simulink model "sistemaPIDSin"  (R2024b)
settings: Solver=VariableStepAuto  StartTime=0.0  StopTime=10  RelTol=1e-3
undefined symbols (not defined in the file): step_value, Ts
settings Model: Creator=estel  LastModifiedBy=estel

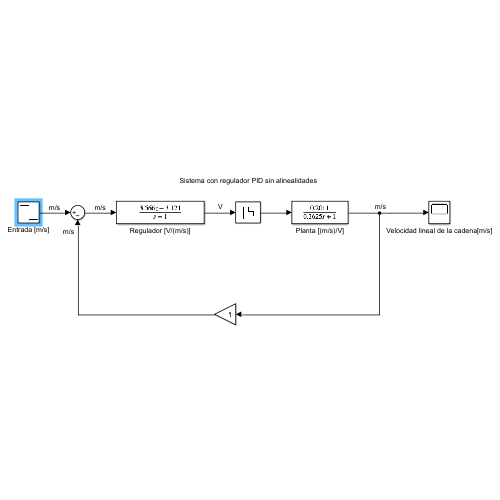
[thumbnail: Simulink's stored preview of the top-level diagram]
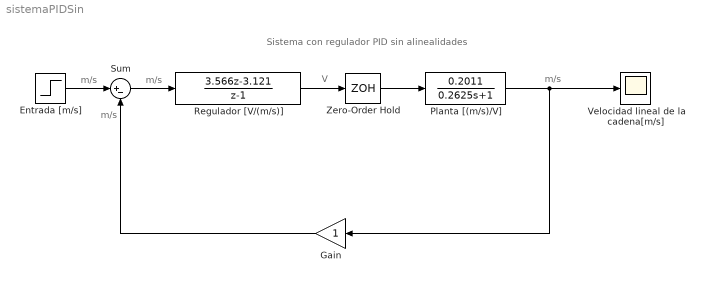
== system sistemaPIDSin ==
  note: m/s
  note: m/s
  note: m/s
  note: m/s
  note: Sistema con regulador PID sin alinealidades
  note: V
  Entrada [m/s] : Step  Time=0  After=step_value  SampleTime=Ts
  Gain : Gain
  Planta [(m/s)/V] : TransferFcn  Numerator=[0.2011]  Denominator=[0.2625 1]
  Regulador [V/(m/s)] : DiscreteTransferFcn  Numerator=[3.566 -3.121]  Denominator=[1 -1]
  Sum : Sum  Inputs=|+-
  Velocidad lineal de la cadena[m/s] : Scope
  Zero-Order Hold : ZeroOrderHold  SampleTime=-1
  wires:
  Planta [(m/s)/V]/1 -> Gain/1, Velocidad lineal de la cadena[m/s]/1
  Entrada [m/s]/1 -> Sum/1
  Sum/1 -> Regulador [V/(m/s)]/1
  Gain/1 -> Sum/2
  Regulador [V/(m/s)]/1 -> Zero-Order Hold/1
  Zero-Order Hold/1 -> Planta [(m/s)/V]/1
